simulink model "Calculator_stateflow"  (R2021a)
settings: Solver=FixedStepDiscrete  StartTime=0.0  StopTime=10.0  RelTol=1e-3  EnableMultiTasking=on
settings Model: Creator=Mina  LastModifiedBy=Mina
settings DataIOCC: ReturnWorkspaceOutputs=off
settings OptimizationCC: DefaultParameterBehavior=Inlined  InlineInvariantSignals=on  EnableMemcpy=off  LifeSpan=1  EfficientTunableParamExpr=on
settings DebuggingCC: UnderspecifiedInitializationDetection=Classic  MergeDetectMultiDrivingBlocksExec=none  SFMachineParentedDataDiag=warning  ArithmeticOperatorsInVariantConditions=warning
settings ModelReferenceCC: PropagateSignalLabelsOutOfModel=off
settings SFSimCC: MATLABDynamicMemAlloc=off  CustomCodeUndefinedFunction=UseInterfaceOnly
settings RTWCC: SystemTargetFile=ert.tlc  GenCodeOnly=on  TemplateMakefile=ert_default_tmf  GenerateReport=on  IncludeHyperlinkInReport=on  LaunchReport=on  GenerateTraceInfo=on  GenerateTraceReport=on  GenerateTraceReportSl=on  GenerateTraceReportSf=on  GenerateTraceReportEml=on
settings CodeAppCC: ForceParamTrailComments=on  IgnoreCustomStorageClasses=off  OperatorAnnotations=on  SimulinkDataObjDesc=on  SFDataObjDesc=on  MATLABFcnDesc=on  InsertBlockDesc=on  StateflowObjectComments=on  MATLABSourceComments=on
settings ERTTargetCC: MultiwordLength=2048  GenerateSampleERTMain=on  InlinedParameterPlacement=NonHierarchical  ERTCustomFileTemplate=example_file_process.tlc

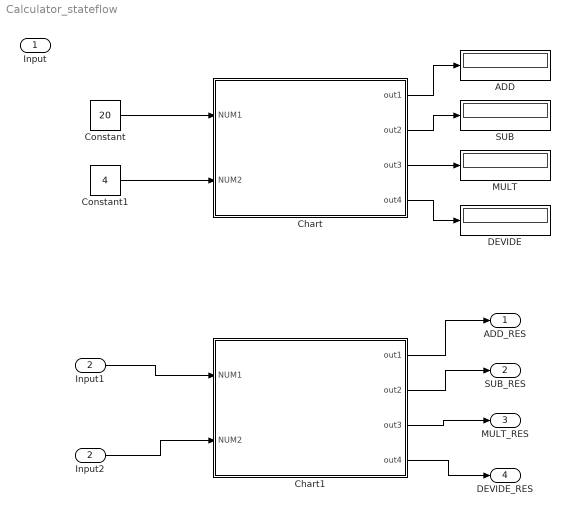
== system Calculator_stateflow ==
  Input : Inport
  Input1 : Inport  Port=2
  ADD : Display
  Chart : Stateflow chart  TreatAsAtomicUnit=on
  Chart1 : Stateflow chart  TreatAsAtomicUnit=on
  Constant : Constant  Value=20  OutDataTypeStr=uint32
  Constant1 : Constant  Value=4  OutDataTypeStr=uint32
  DEVIDE : Display
  Input2 : InportShadow  Port=2
  MULT : Display
  SUB : Display
  ADD_RES : Outport
  SUB_RES : Outport  Port=2
  MULT_RES : Outport  Port=3
  DEVIDE_RES : Outport  Port=4
  wires:
  Constant/1 -> Chart/1(NUM1)
  Constant1/1 -> Chart/2(NUM2)
  Chart/1(out1) -> ADD/1
  Chart/2(out2) -> SUB/1
  Chart/3(out3) -> MULT/1
  Chart/4(out4) -> DEVIDE/1
  Input1/1 -> Chart1/1(NUM1)
  Input2/1 -> Chart1/2(NUM2)
  Chart1/1(out1) -> ADD_RES/1
  Chart1/2(out2) -> SUB_RES/1
  Chart1/3(out3) -> MULT_RES/1
  Chart1/4(out4) -> DEVIDE_RES/1

== stateflow chart Calculator_stateflow/Chart1 ==
  state a=add(b,c) [function]
    (default) -> (junction 2) : {a=b+c;}
  state z=sub(x,y) [function]
    (default) -> (junction 5) : {z=x-y;}
  state k=mult(e,u) [function]
    (default) -> (junction 8) : {k=e*u;}
  state f=devide(w,q) [function]
    (default) -> (junction 11) : {f=w/q;}
  (default) -> (junction 26) : {
      | out1=add(NUM1,NUM2);
      | out2=sub(NUM1,NUM2);
      | out3=mult(NUM1,NUM2);
      | out4=devide(NUM1,NUM2);
      |
      | }
  data: b function_input uint32; c function_input uint32; a function_output uint32; x function_input uint32; y function_input uint32; z function_output uint32; e function_input uint32; u function_input uint32; k function_output uint32; w function_input uint32; q function_input uint32; f function_output uint32; NUM1 input uint32; NUM2 input uint32; out1 output uint32; out2 output uint32; out3 output uint32; out4 output uint32

== stateflow chart Calculator_stateflow/Chart ==
  state a=add(b,c) [function]
    (default) -> (junction 2) : {a=b+c;}
  state z=sub(x,y) [function]
    (default) -> (junction 5) : {z=x-y;}
  state k=mult(e,u) [function]
    (default) -> (junction 8) : {k=e*u;}
  state f=devide(w,q) [function]
    (default) -> (junction 11) : {f=w/q;}
  (default) -> (junction 26) : {
      | out1=add(NUM1,NUM2);
      | out2=sub(NUM1,NUM2);
      | out3=mult(NUM1,NUM2);
      | out4=devide(NUM1,NUM2);
      |
      | }
  data: b function_input uint32; c function_input uint32; a function_output uint32; x function_input uint32; y function_input uint32; z function_output uint32; e function_input uint32; u function_input uint32; k function_output uint32; w function_input uint32; q function_input uint32; f function_output uint32; NUM1 input uint32; NUM2 input uint32; out1 output uint32; out2 output uint32; out3 output uint32; out4 output uint32
